simulink model "BMD_2_backup"  (R2025b)
settings: Solver=FixedStepAuto  StartTime=0.0  StopTime=15  FixedStep=0.005  RelTol=1e-3
values from neighbouring files (symbols this model uses):
  FPV_mass = 0.8    [Soft.m]
  g = 9.81    [Soft.m]
  ks = 0    [Soft.m]
  p_0 = 1013.25    [Soft.m]
  Q2Ts = forcetomotors()    [Soft.m]    (also in forcetomotors.m = inv(Ts2Q))
  takeOffDuration = 2    [Soft.m]
  Ts = 0.005    [Soft.m]
undefined symbols (not defined in the file or in its folder): CdA, DiscIntNeverNeededParam, Dw, kd_dz, kd_pos_dx, kd_pos_dy, kd_pq, kd_pr, kd_y, kd_z, ki_dz, ki_pos_dx, ki_pos_dy, ki_pq, ki_pr, ki_y, ki_z, kp_dz, kp_pos_dx, kp_pos_dy, kp_pos_x, kp_pos_y, kp_pq, kp_pr, kp_y, kp_z, pInitialization, rho
libraries: simulink x43, discretizing x18, slpidlib x3, SignalEditorBlockLib x2, shared6dof x1, dynamicsLibrary x1, aerolibasang x1, aerolibnav x1
(part 9 of 22)

== system BMD_2_backup/FCS/Controller/position_controller/pos_dx_pid/Sum ==
  P : Inport  SampleTime=SampleTime
  I : Inport  Port=2  SampleTime=SampleTime
  D : Inport  Port=3  SampleTime=SampleTime
  Passthrough_I : Subsystem  VariantControl=Passthrough_I
  Passthrough_P : Subsystem  VariantControl=Passthrough_P
  Sum_PD : Subsystem  VariantControl=Sum_PD
  Sum_PI : Subsystem  VariantControl=Sum_PI
  Sum_PID : Subsystem  VariantControl=Sum_PID
  Out1 : Outport  SampleTime=SampleTime

== system BMD_2_backup/FCS/Controller/position_controller/pos_dx_pid/Sum Fdbk ==
  fromP : Inport  SampleTime=SampleTime
  fromState : Inport  Port=2  SampleTime=SampleTime
  fromD : Inport  Port=3  SampleTime=SampleTime
  Disabled : Subsystem  VariantControl=Disabled
  Enabled : Subsystem  VariantControl=Enabled
  Passthrough : Subsystem  VariantControl=Passthrough
  Out1 : Outport  SampleTime=SampleTime

== system BMD_2_backup/FCS/Controller/position_controller/pos_dx_pid/Tracking Mode ==
  uout : Inport  SampleTime=SampleTime
  TR : Inport  Port=2  SampleTime=SampleTime
  Disabled : Subsystem  VariantControl=Disabled
  Enabled : Subsystem  VariantControl=Enabled
  Out1 : Outport  SampleTime=SampleTime

== system BMD_2_backup/FCS/Controller/position_controller/pos_dx_pid/Tracking Mode Sum ==
  fromIgain : Inport  SampleTime=SampleTime
  fromTR : Inport  Port=2  SampleTime=SampleTime
  Passthrough : Subsystem  VariantControl=Passthrough
  Tracking Mode : Subsystem  VariantControl=TrackingMode
  preInt : Outport

== system BMD_2_backup/FCS/Controller/position_controller/pos_dx_pid/Tsamp - Integral ==
  U : Inport  SampleTime=SampleTime
  Ts : Inport  Port=2  SampleTime=SampleTime
  Disabled : Subsystem  VariantControl=Disabled
  External Ts : Subsystem  VariantControl=ExternalTs
  Passthrough : Subsystem  VariantControl=Passthrough
  TsSignalSpecification : Subsystem  VariantControl=Disabled_SignalSpec
  Out1 : Outport  SampleTime=SampleTime

== system BMD_2_backup/FCS/Controller/position_controller/pos_dx_pid/Tsamp - Ngain ==
  U : Inport  SampleTime=SampleTime
  Ts : Inport  Port=2  SampleTime=SampleTime
  External Ts : Subsystem  VariantControl=ExternalTs
  Passthrough : Subsystem  VariantControl=Passthrough
  Out1 : Outport  SampleTime=SampleTime

== system BMD_2_backup/FCS/Controller/position_controller/pos_dx_pid/postSat Signal ==
  feedback : Inport  SampleTime=SampleTime
  forward : Inport  Port=2  SampleTime=SampleTime
  Feedback_Path : Subsystem  VariantControl=Feedback
  Forward_Path : Subsystem  VariantControl=Forward
  Out1 : Outport  SampleTime=SampleTime

== system BMD_2_backup/FCS/Controller/position_controller/pos_dx_pid/preInt Signal ==
  preInt : Inport  SampleTime=SampleTime
  extAW : Inport  Port=2  SampleTime=SampleTime
  External PreInt : Subsystem  VariantControl=ExternalPreInt
  Internal PreInt : Subsystem  VariantControl=InternalPreInt
  Out1 : Outport  SampleTime=SampleTime

== system BMD_2_backup/FCS/Controller/position_controller/pos_dx_pid/preSat Signal ==
  feedback : Inport  SampleTime=SampleTime
  forward : Inport  Port=2  SampleTime=SampleTime
  Feedback_Path : Subsystem  VariantControl=Feedback
  Forward_Path : Subsystem  VariantControl=Forward
  Out1 : Outport  SampleTime=SampleTime

== system BMD_2_backup/FCS/Controller/position_controller/pos_dy_pid/Anti-windup ==
  preSat : Inport  SampleTime=SampleTime
  postSat : Inport  Port=2  SampleTime=SampleTime
  P : Inport  Port=3  SampleTime=SampleTime
  preInt : Inport  Port=4  SampleTime=SampleTime
  Upper Limit : Inport  Port=5  SampleTime=SampleTime
  Lower Limit : Inport  Port=6  SampleTime=SampleTime
  Back Calculation : Subsystem  VariantControl=BackCalculation
  Cont. Clamping Ideal : Subsystem  VariantControl=ContClampingIdeal
  Cont. Clamping Parallel : Subsystem  VariantControl=ContClampingParallel
  Disabled : Subsystem  VariantControl=Disabled
  Disc. Clamping Ideal : Subsystem  VariantControl=DiscClampingIdeal
  Disc. Clamping Parallel : Subsystem  VariantControl=DiscClampingParallel
  Passthrough : Subsystem  VariantControl=Passthrough
  Out1 : Outport  SampleTime=SampleTime

== system BMD_2_backup/FCS/Controller/position_controller/pos_dy_pid/D Gain ==
  err : Inport  SampleTime=SampleTime
  D Gain : Inport  Port=2  SampleTime=SampleTime
  Disabled : Subsystem  VariantControl=Disabled
  External Parameters : Subsystem  VariantControl=ExternalParameters
  Internal Parameters : Subsystem  VariantControl=InternalParameters
  Out1 : Outport  SampleTime=SampleTime

== system BMD_2_backup/FCS/Controller/position_controller/pos_dy_pid/External Derivative ==
  err : Inport  SampleTime=SampleTime
  ydot : Inport  Port=2  SampleTime=SampleTime
  Disabled : Subsystem  VariantControl=Disabled
  Error : Subsystem  VariantControl=ErrorSignal
  External Ydot : Subsystem  VariantControl=ExternalYdot
  Out1 : Outport  SampleTime=SampleTime

== system BMD_2_backup/FCS/Controller/position_controller/pos_dy_pid/Filter ==
  Reset : Inport  SampleTime=SampleTime
  U : Inport  Port=2  SampleTime=SampleTime
  N : Inport  Port=3  SampleTime=SampleTime
  D0in : Inport  Port=4  SampleTime=SampleTime
  Nout : Inport  Port=5  SampleTime=SampleTime
  Ts : Inport  Port=6  SampleTime=SampleTime
  Cont. Filter : Subsystem  VariantControl=ContFilter
  Cont. Filter Only : Subsystem  VariantControl=ContFilterOnly
  Differentiator : Subsystem  VariantControl=Differentiator
  Disabled : Subsystem  VariantControl=Disabled
  Disc. Backward Euler Filter : Subsystem  VariantControl=BackwardEulerFilter
  Disc. Backward Euler Filter Only : Subsystem  VariantControl=BackwardEulerFilterOnly
  Disc. Forward Euler Filter : Subsystem  VariantControl=ForwardEulerFilter
  Disc. Forward Euler Filter Only : Subsystem  VariantControl=ForwardEulerFilterOnly
  Disc. Trapezoidal Filter : Subsystem  VariantControl=TrapezoidalFilter
  Disc. Trapezoidal Filter Only : Subsystem  VariantControl=TrapezoidalFilterOnly
  Passthrough : Subsystem  VariantControl=Passthrough
  Y : Outport  SampleTime=SampleTime

== system BMD_2_backup/FCS/Controller/position_controller/pos_dy_pid/Filter ICs ==
  D0 : Inport  SampleTime=SampleTime
  Disabled : Subsystem  VariantControl=Disabled
  External IC : Subsystem  VariantControl=ExternalICs
  Internal IC - Differentiator : Subsystem  VariantControl=InternalICsDifferentiator
  Internal IC - Filter : Subsystem  VariantControl=InternalICsFilter
  Out1 : Outport  SampleTime=SampleTime

== system BMD_2_backup/FCS/Controller/position_controller/pos_dy_pid/I Gain ==
  err : Inport  SampleTime=SampleTime
  I Gain : Inport  Port=2  SampleTime=SampleTime
  Disabled : Subsystem  VariantControl=Disabled
  External Parameters : Subsystem  VariantControl=ExternalParameters
  Internal Parameters : Subsystem  VariantControl=InternalParameters
  Out1 : Outport  SampleTime=SampleTime

== system BMD_2_backup/FCS/Controller/position_controller/pos_dy_pid/Ideal P Gain ==
  In1 : Inport  SampleTime=SampleTime
  P Gain : Inport  Port=2  SampleTime=SampleTime
  External Parameters : Subsystem  VariantControl=ExternalParameters
  Internal Parameters : Subsystem  VariantControl=InternalParameters
  Passthrough : Subsystem  VariantControl=Disabled
  Out1 : Outport  SampleTime=SampleTime

== system BMD_2_backup/FCS/Controller/position_controller/pos_dy_pid/Ideal P Gain Fdbk ==
  In1 : Inport  SampleTime=SampleTime
  P Gain : Inport  Port=2  SampleTime=SampleTime
  Disabled : Subsystem  VariantControl=Disabled
  External Parameters : Subsystem  VariantControl=ExternalParameters
  Internal Parameters : Subsystem  VariantControl=InternalParameters
  Passthrough : Subsystem  VariantControl=Passthrough
  Out1 : Outport  SampleTime=SampleTime

== system BMD_2_backup/FCS/Controller/position_controller/pos_dy_pid/Integrator ==
  U : Inport  SampleTime=SampleTime
  I0in : Inport  Port=2  SampleTime=SampleTime
  Reset : Inport  Port=3  SampleTime=SampleTime
  Continuous : Subsystem  VariantControl=Continuous
  Disabled : Subsystem  VariantControl=Disabled
  Discrete : Subsystem  VariantControl=Discrete
  state : Outport  SampleTime=SampleTime
  out : Outport  Port=2  SampleTime=SampleTime

== system BMD_2_backup/FCS/Controller/position_controller/pos_dy_pid/Integrator ICs ==
  I0 : Inport  SampleTime=SampleTime
  Disabled : Subsystem  VariantControl=Disabled
  External IC : Subsystem  VariantControl=ExternalICs
  Internal IC : Subsystem  VariantControl=InternalICs
  Out1 : Outport  SampleTime=SampleTime

== system BMD_2_backup/FCS/Controller/position_controller/pos_dy_pid/N Copy ==
  N Gain : Inport  SampleTime=SampleTime
  Disabled : Subsystem  VariantControl=Disabled
  Disabled wSignal Specification : Subsystem  VariantControl=Disabled_SignalSpec
  External Parameters : Subsystem  VariantControl=ExternalParameters
  Internal Parameters : Subsystem  VariantControl=InternalParameters
  Out1 : Outport  SampleTime=SampleTime

== system BMD_2_backup/FCS/Controller/position_controller/pos_dy_pid/N Gain ==
  U : Inport  SampleTime=SampleTime
  N Gain : Inport  Port=2  SampleTime=SampleTime
  Disabled : Subsystem  VariantControl=Disabled
  External Parameters : Subsystem  VariantControl=ExternalParameters
  Internal Parameters : Subsystem  VariantControl=InternalParameters
  Passthrough : Subsystem  VariantControl=Passthrough
  Out1 : Outport  SampleTime=SampleTime

== system BMD_2_backup/FCS/Controller/position_controller/pos_dy_pid/P Copy ==
  P Gain : Inport  SampleTime=SampleTime
  Disabled : Subsystem  VariantControl=Disabled
  External Parameters Ideal : Subsystem  VariantControl=ExternalParamsIdeal
  Internal Parameters Ideal : Subsystem  VariantControl=InternalParamsIdeal
  Out1 : Outport  SampleTime=SampleTime

== system BMD_2_backup/FCS/Controller/position_controller/pos_dy_pid/PID Compensator Formula ==

== system BMD_2_backup/FCS/Controller/position_controller/pos_dy_pid/Parallel P Gain ==
  err : Inport  SampleTime=SampleTime
  P Gain : Inport  Port=2  SampleTime=SampleTime
  Disabled : Subsystem  VariantControl=Disabled
  External Parameters : Subsystem  VariantControl=ExternalParameters
  Internal Parameters : Subsystem  VariantControl=InternalParameters
  Passthrough : Subsystem  VariantControl=Passthrough
  Out1 : Outport  SampleTime=SampleTime

== system BMD_2_backup/FCS/Controller/position_controller/pos_dy_pid/Reset Signal ==
  Reset : Inport  SampleTime=SampleTime
  Disabled : Subsystem  VariantControl=Disabled
  External Reset : Subsystem  VariantControl=ExternalReset
  Out1 : Outport  SampleTime=SampleTime

== system BMD_2_backup/FCS/Controller/position_controller/pos_dy_pid/Saturation ==
  In1 : Inport  SampleTime=SampleTime
  Upper Limit : Inport  Port=2  SampleTime=SampleTime
  Lower Limit : Inport  Port=3  SampleTime=SampleTime
  Enabled : Subsystem  VariantControl=Enabled
  External : Subsystem  VariantControl=External
  Passthrough : Subsystem  VariantControl=Disabled
  Out1 : Outport  SampleTime=SampleTime

== system BMD_2_backup/FCS/Controller/position_controller/pos_dy_pid/Saturation Fdbk ==
  In1 : Inport  SampleTime=SampleTime
  Upper Limit : Inport  Port=2  SampleTime=SampleTime
  Lower Limit : Inport  Port=3  SampleTime=SampleTime
  Disabled : Subsystem  VariantControl=Disabled
  Enabled : Subsystem  VariantControl=Enabled
  External : Subsystem  VariantControl=External
  Passthrough : Subsystem  VariantControl=Passthrough
  Out1 : Outport  SampleTime=SampleTime

== system BMD_2_backup/FCS/Controller/position_controller/pos_dy_pid/Sum ==
  P : Inport  SampleTime=SampleTime
  I : Inport  Port=2  SampleTime=SampleTime
  D : Inport  Port=3  SampleTime=SampleTime
  Passthrough_I : Subsystem  VariantControl=Passthrough_I
  Passthrough_P : Subsystem  VariantControl=Passthrough_P
  Sum_PD : Subsystem  VariantControl=Sum_PD
  Sum_PI : Subsystem  VariantControl=Sum_PI
  Sum_PID : Subsystem  VariantControl=Sum_PID
  Out1 : Outport  SampleTime=SampleTime

== system BMD_2_backup/FCS/Controller/position_controller/pos_dy_pid/Sum Fdbk ==
  fromP : Inport  SampleTime=SampleTime
  fromState : Inport  Port=2  SampleTime=SampleTime
  fromD : Inport  Port=3  SampleTime=SampleTime
  Disabled : Subsystem  VariantControl=Disabled
  Enabled : Subsystem  VariantControl=Enabled
  Passthrough : Subsystem  VariantControl=Passthrough
  Out1 : Outport  SampleTime=SampleTime

== system BMD_2_backup/FCS/Controller/position_controller/pos_dy_pid/Tracking Mode ==
  uout : Inport  SampleTime=SampleTime
  TR : Inport  Port=2  SampleTime=SampleTime
  Disabled : Subsystem  VariantControl=Disabled
  Enabled : Subsystem  VariantControl=Enabled
  Out1 : Outport  SampleTime=SampleTime

== system BMD_2_backup/FCS/Controller/position_controller/pos_dy_pid/Tracking Mode Sum ==
  fromIgain : Inport  SampleTime=SampleTime
  fromTR : Inport  Port=2  SampleTime=SampleTime
  Passthrough : Subsystem  VariantControl=Passthrough
  Tracking Mode : Subsystem  VariantControl=TrackingMode
  preInt : Outport

== system BMD_2_backup/FCS/Controller/position_controller/pos_dy_pid/Tsamp - Integral ==
  U : Inport  SampleTime=SampleTime
  Ts : Inport  Port=2  SampleTime=SampleTime
  Disabled : Subsystem  VariantControl=Disabled
  External Ts : Subsystem  VariantControl=ExternalTs
  Passthrough : Subsystem  VariantControl=Passthrough
  TsSignalSpecification : Subsystem  VariantControl=Disabled_SignalSpec
  Out1 : Outport  SampleTime=SampleTime

== system BMD_2_backup/FCS/Controller/position_controller/pos_dy_pid/Tsamp - Ngain ==
  U : Inport  SampleTime=SampleTime
  Ts : Inport  Port=2  SampleTime=SampleTime
  External Ts : Subsystem  VariantControl=ExternalTs
  Passthrough : Subsystem  VariantControl=Passthrough
  Out1 : Outport  SampleTime=SampleTime

== system BMD_2_backup/FCS/Controller/position_controller/pos_dy_pid/postSat Signal ==
  feedback : Inport  SampleTime=SampleTime
  forward : Inport  Port=2  SampleTime=SampleTime
  Feedback_Path : Subsystem  VariantControl=Feedback
  Forward_Path : Subsystem  VariantControl=Forward
  Out1 : Outport  SampleTime=SampleTime

== system BMD_2_backup/FCS/Controller/position_controller/pos_dy_pid/preInt Signal ==
  preInt : Inport  SampleTime=SampleTime
  extAW : Inport  Port=2  SampleTime=SampleTime
  External PreInt : Subsystem  VariantControl=ExternalPreInt
  Internal PreInt : Subsystem  VariantControl=InternalPreInt
  Out1 : Outport  SampleTime=SampleTime

== system BMD_2_backup/FCS/Controller/position_controller/pos_dy_pid/preSat Signal ==
  feedback : Inport  SampleTime=SampleTime
  forward : Inport  Port=2  SampleTime=SampleTime
  Feedback_Path : Subsystem  VariantControl=Feedback
  Forward_Path : Subsystem  VariantControl=Forward
  Out1 : Outport  SampleTime=SampleTime

== system BMD_2_backup/FCS/Controller/position_controller/pos_x_pid/Anti-windup ==
  preSat : Inport  SampleTime=SampleTime
  postSat : Inport  Port=2  SampleTime=SampleTime
  P : Inport  Port=3  SampleTime=SampleTime
  preInt : Inport  Port=4  SampleTime=SampleTime
  Upper Limit : Inport  Port=5  SampleTime=SampleTime
  Lower Limit : Inport  Port=6  SampleTime=SampleTime
  Back Calculation : Subsystem  VariantControl=BackCalculation
  Cont. Clamping Ideal : Subsystem  VariantControl=ContClampingIdeal
  Cont. Clamping Parallel : Subsystem  VariantControl=ContClampingParallel
  Disabled : Subsystem  VariantControl=Disabled
  Disc. Clamping Ideal : Subsystem  VariantControl=DiscClampingIdeal
  Disc. Clamping Parallel : Subsystem  VariantControl=DiscClampingParallel
  Passthrough : Subsystem  VariantControl=Passthrough
  Out1 : Outport  SampleTime=SampleTime

== system BMD_2_backup/FCS/Controller/position_controller/pos_x_pid/D Gain ==
  err : Inport  SampleTime=SampleTime
  D Gain : Inport  Port=2  SampleTime=SampleTime
  Disabled : Subsystem  VariantControl=Disabled
  External Parameters : Subsystem  VariantControl=ExternalParameters
  Internal Parameters : Subsystem  VariantControl=InternalParameters
  Out1 : Outport  SampleTime=SampleTime

== system BMD_2_backup/FCS/Controller/position_controller/pos_x_pid/External Derivative ==
  err : Inport  SampleTime=SampleTime
  ydot : Inport  Port=2  SampleTime=SampleTime
  Disabled : Subsystem  VariantControl=Disabled
  Error : Subsystem  VariantControl=ErrorSignal
  External Ydot : Subsystem  VariantControl=ExternalYdot
  Out1 : Outport  SampleTime=SampleTime

== system BMD_2_backup/FCS/Controller/position_controller/pos_x_pid/Filter ==
  Reset : Inport  SampleTime=SampleTime
  U : Inport  Port=2  SampleTime=SampleTime
  N : Inport  Port=3  SampleTime=SampleTime
  D0in : Inport  Port=4  SampleTime=SampleTime
  Nout : Inport  Port=5  SampleTime=SampleTime
  Ts : Inport  Port=6  SampleTime=SampleTime
  Cont. Filter : Subsystem  VariantControl=ContFilter
  Cont. Filter Only : Subsystem  VariantControl=ContFilterOnly
  Differentiator : Subsystem  VariantControl=Differentiator
  Disabled : Subsystem  VariantControl=Disabled
  Disc. Backward Euler Filter : Subsystem  VariantControl=BackwardEulerFilter
  Disc. Backward Euler Filter Only : Subsystem  VariantControl=BackwardEulerFilterOnly
  Disc. Forward Euler Filter : Subsystem  VariantControl=ForwardEulerFilter
  Disc. Forward Euler Filter Only : Subsystem  VariantControl=ForwardEulerFilterOnly
  Disc. Trapezoidal Filter : Subsystem  VariantControl=TrapezoidalFilter
  Disc. Trapezoidal Filter Only : Subsystem  VariantControl=TrapezoidalFilterOnly
  Passthrough : Subsystem  VariantControl=Passthrough
  Y : Outport  SampleTime=SampleTime

== system BMD_2_backup/FCS/Controller/position_controller/pos_x_pid/Filter ICs ==
  D0 : Inport  SampleTime=SampleTime
  Disabled : Subsystem  VariantControl=Disabled
  External IC : Subsystem  VariantControl=ExternalICs
  Internal IC - Differentiator : Subsystem  VariantControl=InternalICsDifferentiator
  Internal IC - Filter : Subsystem  VariantControl=InternalICsFilter
  Out1 : Outport  SampleTime=SampleTime

== system BMD_2_backup/FCS/Controller/position_controller/pos_x_pid/I Gain ==
  err : Inport  SampleTime=SampleTime
  I Gain : Inport  Port=2  SampleTime=SampleTime
  Disabled : Subsystem  VariantControl=Disabled
  External Parameters : Subsystem  VariantControl=ExternalParameters
  Internal Parameters : Subsystem  VariantControl=InternalParameters
  Out1 : Outport  SampleTime=SampleTime

== system BMD_2_backup/FCS/Controller/position_controller/pos_x_pid/Ideal P Gain ==
  In1 : Inport  SampleTime=SampleTime
  P Gain : Inport  Port=2  SampleTime=SampleTime
  External Parameters : Subsystem  VariantControl=ExternalParameters
  Internal Parameters : Subsystem  VariantControl=InternalParameters
  Passthrough : Subsystem  VariantControl=Disabled
  Out1 : Outport  SampleTime=SampleTime

== system BMD_2_backup/FCS/Controller/position_controller/pos_x_pid/Ideal P Gain Fdbk ==
  In1 : Inport  SampleTime=SampleTime
  P Gain : Inport  Port=2  SampleTime=SampleTime
  Disabled : Subsystem  VariantControl=Disabled
  External Parameters : Subsystem  VariantControl=ExternalParameters
  Internal Parameters : Subsystem  VariantControl=InternalParameters
  Passthrough : Subsystem  VariantControl=Passthrough
  Out1 : Outport  SampleTime=SampleTime

== system BMD_2_backup/FCS/Controller/position_controller/pos_x_pid/Integrator ==
  U : Inport  SampleTime=SampleTime
  I0in : Inport  Port=2  SampleTime=SampleTime
  Reset : Inport  Port=3  SampleTime=SampleTime
  Continuous : Subsystem  VariantControl=Continuous
  Disabled : Subsystem  VariantControl=Disabled
  Discrete : Subsystem  VariantControl=Discrete
  state : Outport  SampleTime=SampleTime
  out : Outport  Port=2  SampleTime=SampleTime

== system BMD_2_backup/FCS/Controller/position_controller/pos_x_pid/Integrator ICs ==
  I0 : Inport  SampleTime=SampleTime
  Disabled : Subsystem  VariantControl=Disabled
  External IC : Subsystem  VariantControl=ExternalICs
  Internal IC : Subsystem  VariantControl=InternalICs
  Out1 : Outport  SampleTime=SampleTime

== system BMD_2_backup/FCS/Controller/position_controller/pos_x_pid/N Copy ==
  N Gain : Inport  SampleTime=SampleTime
  Disabled : Subsystem  VariantControl=Disabled
  Disabled wSignal Specification : Subsystem  VariantControl=Disabled_SignalSpec
  External Parameters : Subsystem  VariantControl=ExternalParameters
  Internal Parameters : Subsystem  VariantControl=InternalParameters
  Out1 : Outport  SampleTime=SampleTime

== system BMD_2_backup/FCS/Controller/position_controller/pos_x_pid/N Gain ==
  U : Inport  SampleTime=SampleTime
  N Gain : Inport  Port=2  SampleTime=SampleTime
  Disabled : Subsystem  VariantControl=Disabled
  External Parameters : Subsystem  VariantControl=ExternalParameters
  Internal Parameters : Subsystem  VariantControl=InternalParameters
  Passthrough : Subsystem  VariantControl=Passthrough
  Out1 : Outport  SampleTime=SampleTime

== system BMD_2_backup/FCS/Controller/position_controller/pos_x_pid/P Copy ==
  P Gain : Inport  SampleTime=SampleTime
  Disabled : Subsystem  VariantControl=Disabled
  External Parameters Ideal : Subsystem  VariantControl=ExternalParamsIdeal
  Internal Parameters Ideal : Subsystem  VariantControl=InternalParamsIdeal
  Out1 : Outport  SampleTime=SampleTime

== system BMD_2_backup/FCS/Controller/position_controller/pos_x_pid/PID Compensator Formula ==

== system BMD_2_backup/FCS/Controller/position_controller/pos_x_pid/Parallel P Gain ==
  err : Inport  SampleTime=SampleTime
  P Gain : Inport  Port=2  SampleTime=SampleTime
  Disabled : Subsystem  VariantControl=Disabled
  External Parameters : Subsystem  VariantControl=ExternalParameters
  Internal Parameters : Subsystem  VariantControl=InternalParameters
  Passthrough : Subsystem  VariantControl=Passthrough
  Out1 : Outport  SampleTime=SampleTime

== system BMD_2_backup/FCS/Controller/position_controller/pos_x_pid/Reset Signal ==
  Reset : Inport  SampleTime=SampleTime
  Disabled : Subsystem  VariantControl=Disabled
  External Reset : Subsystem  VariantControl=ExternalReset
  Out1 : Outport  SampleTime=SampleTime

== system BMD_2_backup/FCS/Controller/position_controller/pos_x_pid/Saturation ==
  In1 : Inport  SampleTime=SampleTime
  Upper Limit : Inport  Port=2  SampleTime=SampleTime
  Lower Limit : Inport  Port=3  SampleTime=SampleTime
  Enabled : Subsystem  VariantControl=Enabled
  External : Subsystem  VariantControl=External
  Passthrough : Subsystem  VariantControl=Disabled
  Out1 : Outport  SampleTime=SampleTime

== system BMD_2_backup/FCS/Controller/position_controller/pos_x_pid/Saturation Fdbk ==
  In1 : Inport  SampleTime=SampleTime
  Upper Limit : Inport  Port=2  SampleTime=SampleTime
  Lower Limit : Inport  Port=3  SampleTime=SampleTime
  Disabled : Subsystem  VariantControl=Disabled
  Enabled : Subsystem  VariantControl=Enabled
  External : Subsystem  VariantControl=External
  Passthrough : Subsystem  VariantControl=Passthrough
  Out1 : Outport  SampleTime=SampleTime

== system BMD_2_backup/FCS/Controller/position_controller/pos_x_pid/Sum ==
  P : Inport  SampleTime=SampleTime
  I : Inport  Port=2  SampleTime=SampleTime
  D : Inport  Port=3  SampleTime=SampleTime
  Passthrough_I : Subsystem  VariantControl=Passthrough_I
  Passthrough_P : Subsystem  VariantControl=Passthrough_P
  Sum_PD : Subsystem  VariantControl=Sum_PD
  Sum_PI : Subsystem  VariantControl=Sum_PI
  Sum_PID : Subsystem  VariantControl=Sum_PID
  Out1 : Outport  SampleTime=SampleTime

== system BMD_2_backup/FCS/Controller/position_controller/pos_x_pid/Sum Fdbk ==
  fromP : Inport  SampleTime=SampleTime
  fromState : Inport  Port=2  SampleTime=SampleTime
  fromD : Inport  Port=3  SampleTime=SampleTime
  Disabled : Subsystem  VariantControl=Disabled
  Enabled : Subsystem  VariantControl=Enabled
  Passthrough : Subsystem  VariantControl=Passthrough
  Out1 : Outport  SampleTime=SampleTime

== system BMD_2_backup/FCS/Controller/position_controller/pos_x_pid/Tracking Mode ==
  uout : Inport  SampleTime=SampleTime
  TR : Inport  Port=2  SampleTime=SampleTime
  Disabled : Subsystem  VariantControl=Disabled
  Enabled : Subsystem  VariantControl=Enabled
  Out1 : Outport  SampleTime=SampleTime

== system BMD_2_backup/FCS/Controller/position_controller/pos_x_pid/Tracking Mode Sum ==
  fromIgain : Inport  SampleTime=SampleTime
  fromTR : Inport  Port=2  SampleTime=SampleTime
  Passthrough : Subsystem  VariantControl=Passthrough
  Tracking Mode : Subsystem  VariantControl=TrackingMode
  preInt : Outport

== system BMD_2_backup/FCS/Controller/position_controller/pos_x_pid/Tsamp - Integral ==
  U : Inport  SampleTime=SampleTime
  Ts : Inport  Port=2  SampleTime=SampleTime
  Disabled : Subsystem  VariantControl=Disabled
  External Ts : Subsystem  VariantControl=ExternalTs
  Passthrough : Subsystem  VariantControl=Passthrough
  TsSignalSpecification : Subsystem  VariantControl=Disabled_SignalSpec
  Out1 : Outport  SampleTime=SampleTime

== system BMD_2_backup/FCS/Controller/position_controller/pos_x_pid/Tsamp - Ngain ==
  U : Inport  SampleTime=SampleTime
  Ts : Inport  Port=2  SampleTime=SampleTime
  External Ts : Subsystem  VariantControl=ExternalTs
  Passthrough : Subsystem  VariantControl=Passthrough
  Out1 : Outport  SampleTime=SampleTime

== system BMD_2_backup/FCS/Controller/position_controller/pos_x_pid/postSat Signal ==
  feedback : Inport  SampleTime=SampleTime
  forward : Inport  Port=2  SampleTime=SampleTime
  Feedback_Path : Subsystem  VariantControl=Feedback
  Forward_Path : Subsystem  VariantControl=Forward
  Out1 : Outport  SampleTime=SampleTime

== system BMD_2_backup/FCS/Controller/position_controller/pos_x_pid/preInt Signal ==
  preInt : Inport  SampleTime=SampleTime
  extAW : Inport  Port=2  SampleTime=SampleTime
  External PreInt : Subsystem  VariantControl=ExternalPreInt
  Internal PreInt : Subsystem  VariantControl=InternalPreInt
  Out1 : Outport  SampleTime=SampleTime

== system BMD_2_backup/FCS/Controller/position_controller/pos_x_pid/preSat Signal ==
  feedback : Inport  SampleTime=SampleTime
  forward : Inport  Port=2  SampleTime=SampleTime
  Feedback_Path : Subsystem  VariantControl=Feedback
  Forward_Path : Subsystem  VariantControl=Forward
  Out1 : Outport  SampleTime=SampleTime

== system BMD_2_backup/FCS/Controller/position_controller/pos_y_pid/Anti-windup ==
  preSat : Inport  SampleTime=SampleTime
  postSat : Inport  Port=2  SampleTime=SampleTime
  P : Inport  Port=3  SampleTime=SampleTime
  preInt : Inport  Port=4  SampleTime=SampleTime
  Upper Limit : Inport  Port=5  SampleTime=SampleTime
  Lower Limit : Inport  Port=6  SampleTime=SampleTime
  Back Calculation : Subsystem  VariantControl=BackCalculation
  Cont. Clamping Ideal : Subsystem  VariantControl=ContClampingIdeal
  Cont. Clamping Parallel : Subsystem  VariantControl=ContClampingParallel
  Disabled : Subsystem  VariantControl=Disabled
  Disc. Clamping Ideal : Subsystem  VariantControl=DiscClampingIdeal
  Disc. Clamping Parallel : Subsystem  VariantControl=DiscClampingParallel
  Passthrough : Subsystem  VariantControl=Passthrough
  Out1 : Outport  SampleTime=SampleTime

== system BMD_2_backup/FCS/Controller/position_controller/pos_y_pid/D Gain ==
  err : Inport  SampleTime=SampleTime
  D Gain : Inport  Port=2  SampleTime=SampleTime
  Disabled : Subsystem  VariantControl=Disabled
  External Parameters : Subsystem  VariantControl=ExternalParameters
  Internal Parameters : Subsystem  VariantControl=InternalParameters
  Out1 : Outport  SampleTime=SampleTime

== system BMD_2_backup/FCS/Controller/position_controller/pos_y_pid/External Derivative ==
  err : Inport  SampleTime=SampleTime
  ydot : Inport  Port=2  SampleTime=SampleTime
  Disabled : Subsystem  VariantControl=Disabled
  Error : Subsystem  VariantControl=ErrorSignal
  External Ydot : Subsystem  VariantControl=ExternalYdot
  Out1 : Outport  SampleTime=SampleTime

== system BMD_2_backup/FCS/Controller/position_controller/pos_y_pid/Filter ==
  Reset : Inport  SampleTime=SampleTime
  U : Inport  Port=2  SampleTime=SampleTime
  N : Inport  Port=3  SampleTime=SampleTime
  D0in : Inport  Port=4  SampleTime=SampleTime
  Nout : Inport  Port=5  SampleTime=SampleTime
  Ts : Inport  Port=6  SampleTime=SampleTime
  Cont. Filter : Subsystem  VariantControl=ContFilter
  Cont. Filter Only : Subsystem  VariantControl=ContFilterOnly
  Differentiator : Subsystem  VariantControl=Differentiator
  Disabled : Subsystem  VariantControl=Disabled
  Disc. Backward Euler Filter : Subsystem  VariantControl=BackwardEulerFilter
  Disc. Backward Euler Filter Only : Subsystem  VariantControl=BackwardEulerFilterOnly
  Disc. Forward Euler Filter : Subsystem  VariantControl=ForwardEulerFilter
  Disc. Forward Euler Filter Only : Subsystem  VariantControl=ForwardEulerFilterOnly
  Disc. Trapezoidal Filter : Subsystem  VariantControl=TrapezoidalFilter
  Disc. Trapezoidal Filter Only : Subsystem  VariantControl=TrapezoidalFilterOnly
  Passthrough : Subsystem  VariantControl=Passthrough
  Y : Outport  SampleTime=SampleTime

== system BMD_2_backup/FCS/Controller/position_controller/pos_y_pid/Filter ICs ==
  D0 : Inport  SampleTime=SampleTime
  Disabled : Subsystem  VariantControl=Disabled
  External IC : Subsystem  VariantControl=ExternalICs
  Internal IC - Differentiator : Subsystem  VariantControl=InternalICsDifferentiator
  Internal IC - Filter : Subsystem  VariantControl=InternalICsFilter
  Out1 : Outport  SampleTime=SampleTime

== system BMD_2_backup/FCS/Controller/position_controller/pos_y_pid/I Gain ==
  err : Inport  SampleTime=SampleTime
  I Gain : Inport  Port=2  SampleTime=SampleTime
  Disabled : Subsystem  VariantControl=Disabled
  External Parameters : Subsystem  VariantControl=ExternalParameters
  Internal Parameters : Subsystem  VariantControl=InternalParameters
  Out1 : Outport  SampleTime=SampleTime

== system BMD_2_backup/FCS/Controller/position_controller/pos_y_pid/Ideal P Gain ==
  In1 : Inport  SampleTime=SampleTime
  P Gain : Inport  Port=2  SampleTime=SampleTime
  External Parameters : Subsystem  VariantControl=ExternalParameters
  Internal Parameters : Subsystem  VariantControl=InternalParameters
  Passthrough : Subsystem  VariantControl=Disabled
  Out1 : Outport  SampleTime=SampleTime

== system BMD_2_backup/FCS/Controller/position_controller/pos_y_pid/Ideal P Gain Fdbk ==
  In1 : Inport  SampleTime=SampleTime
  P Gain : Inport  Port=2  SampleTime=SampleTime
  Disabled : Subsystem  VariantControl=Disabled
  External Parameters : Subsystem  VariantControl=ExternalParameters
  Internal Parameters : Subsystem  VariantControl=InternalParameters
  Passthrough : Subsystem  VariantControl=Passthrough
  Out1 : Outport  SampleTime=SampleTime

== system BMD_2_backup/FCS/Controller/position_controller/pos_y_pid/Integrator ==
  U : Inport  SampleTime=SampleTime
  I0in : Inport  Port=2  SampleTime=SampleTime
  Reset : Inport  Port=3  SampleTime=SampleTime
  Continuous : Subsystem  VariantControl=Continuous
  Disabled : Subsystem  VariantControl=Disabled
  Discrete : Subsystem  VariantControl=Discrete
  state : Outport  SampleTime=SampleTime
  out : Outport  Port=2  SampleTime=SampleTime

== system BMD_2_backup/FCS/Controller/position_controller/pos_y_pid/Integrator ICs ==
  I0 : Inport  SampleTime=SampleTime
  Disabled : Subsystem  VariantControl=Disabled
  External IC : Subsystem  VariantControl=ExternalICs
  Internal IC : Subsystem  VariantControl=InternalICs
  Out1 : Outport  SampleTime=SampleTime

== system BMD_2_backup/FCS/Controller/position_controller/pos_y_pid/N Copy ==
  N Gain : Inport  SampleTime=SampleTime
  Disabled : Subsystem  VariantControl=Disabled
  Disabled wSignal Specification : Subsystem  VariantControl=Disabled_SignalSpec
  External Parameters : Subsystem  VariantControl=ExternalParameters
  Internal Parameters : Subsystem  VariantControl=InternalParameters
  Out1 : Outport  SampleTime=SampleTime

== system BMD_2_backup/FCS/Controller/position_controller/pos_y_pid/N Gain ==
  U : Inport  SampleTime=SampleTime
  N Gain : Inport  Port=2  SampleTime=SampleTime
  Disabled : Subsystem  VariantControl=Disabled
  External Parameters : Subsystem  VariantControl=ExternalParameters
  Internal Parameters : Subsystem  VariantControl=InternalParameters
  Passthrough : Subsystem  VariantControl=Passthrough
  Out1 : Outport  SampleTime=SampleTime

== system BMD_2_backup/FCS/Controller/position_controller/pos_y_pid/P Copy ==
  P Gain : Inport  SampleTime=SampleTime
  Disabled : Subsystem  VariantControl=Disabled
  External Parameters Ideal : Subsystem  VariantControl=ExternalParamsIdeal
  Internal Parameters Ideal : Subsystem  VariantControl=InternalParamsIdeal
  Out1 : Outport  SampleTime=SampleTime

== system BMD_2_backup/FCS/Controller/position_controller/pos_y_pid/PID Compensator Formula ==

== system BMD_2_backup/FCS/Controller/position_controller/pos_y_pid/Parallel P Gain ==
  err : Inport  SampleTime=SampleTime
  P Gain : Inport  Port=2  SampleTime=SampleTime
  Disabled : Subsystem  VariantControl=Disabled
  External Parameters : Subsystem  VariantControl=ExternalParameters
  Internal Parameters : Subsystem  VariantControl=InternalParameters
  Passthrough : Subsystem  VariantControl=Passthrough
  Out1 : Outport  SampleTime=SampleTime

== system BMD_2_backup/FCS/Controller/position_controller/pos_y_pid/Reset Signal ==
  Reset : Inport  SampleTime=SampleTime
  Disabled : Subsystem  VariantControl=Disabled
  External Reset : Subsystem  VariantControl=ExternalReset
  Out1 : Outport  SampleTime=SampleTime

== system BMD_2_backup/FCS/Controller/position_controller/pos_y_pid/Saturation ==
  In1 : Inport  SampleTime=SampleTime
  Upper Limit : Inport  Port=2  SampleTime=SampleTime
  Lower Limit : Inport  Port=3  SampleTime=SampleTime
  Enabled : Subsystem  VariantControl=Enabled
  External : Subsystem  VariantControl=External
  Passthrough : Subsystem  VariantControl=Disabled
  Out1 : Outport  SampleTime=SampleTime

== system BMD_2_backup/FCS/Controller/position_controller/pos_y_pid/Saturation Fdbk ==
  In1 : Inport  SampleTime=SampleTime
  Upper Limit : Inport  Port=2  SampleTime=SampleTime
  Lower Limit : Inport  Port=3  SampleTime=SampleTime
  Disabled : Subsystem  VariantControl=Disabled
  Enabled : Subsystem  VariantControl=Enabled
  External : Subsystem  VariantControl=External
  Passthrough : Subsystem  VariantControl=Passthrough
  Out1 : Outport  SampleTime=SampleTime

== system BMD_2_backup/FCS/Controller/position_controller/pos_y_pid/Sum ==
  P : Inport  SampleTime=SampleTime
  I : Inport  Port=2  SampleTime=SampleTime
  D : Inport  Port=3  SampleTime=SampleTime
  Passthrough_I : Subsystem  VariantControl=Passthrough_I
  Passthrough_P : Subsystem  VariantControl=Passthrough_P
  Sum_PD : Subsystem  VariantControl=Sum_PD
  Sum_PI : Subsystem  VariantControl=Sum_PI
  Sum_PID : Subsystem  VariantControl=Sum_PID
  Out1 : Outport  SampleTime=SampleTime

== system BMD_2_backup/FCS/Controller/position_controller/pos_y_pid/Sum Fdbk ==
  fromP : Inport  SampleTime=SampleTime
  fromState : Inport  Port=2  SampleTime=SampleTime
  fromD : Inport  Port=3  SampleTime=SampleTime
  Disabled : Subsystem  VariantControl=Disabled
  Enabled : Subsystem  VariantControl=Enabled
  Passthrough : Subsystem  VariantControl=Passthrough
  Out1 : Outport  SampleTime=SampleTime

== system BMD_2_backup/FCS/Controller/position_controller/pos_y_pid/Tracking Mode ==
  uout : Inport  SampleTime=SampleTime
  TR : Inport  Port=2  SampleTime=SampleTime
  Disabled : Subsystem  VariantControl=Disabled
  Enabled : Subsystem  VariantControl=Enabled
  Out1 : Outport  SampleTime=SampleTime

== system BMD_2_backup/FCS/Controller/position_controller/pos_y_pid/Tracking Mode Sum ==
  fromIgain : Inport  SampleTime=SampleTime
  fromTR : Inport  Port=2  SampleTime=SampleTime
  Passthrough : Subsystem  VariantControl=Passthrough
  Tracking Mode : Subsystem  VariantControl=TrackingMode
  preInt : Outport

== system BMD_2_backup/FCS/Controller/position_controller/pos_y_pid/Tsamp - Integral ==
  U : Inport  SampleTime=SampleTime
  Ts : Inport  Port=2  SampleTime=SampleTime
  Disabled : Subsystem  VariantControl=Disabled
  External Ts : Subsystem  VariantControl=ExternalTs
  Passthrough : Subsystem  VariantControl=Passthrough
  TsSignalSpecification : Subsystem  VariantControl=Disabled_SignalSpec
  Out1 : Outport  SampleTime=SampleTime

== system BMD_2_backup/FCS/Controller/position_controller/pos_y_pid/Tsamp - Ngain ==
  U : Inport  SampleTime=SampleTime
  Ts : Inport  Port=2  SampleTime=SampleTime
  External Ts : Subsystem  VariantControl=ExternalTs
  Passthrough : Subsystem  VariantControl=Passthrough
  Out1 : Outport  SampleTime=SampleTime

== system BMD_2_backup/FCS/Controller/position_controller/pos_y_pid/postSat Signal ==
  feedback : Inport  SampleTime=SampleTime
  forward : Inport  Port=2  SampleTime=SampleTime
  Feedback_Path : Subsystem  VariantControl=Feedback
  Forward_Path : Subsystem  VariantControl=Forward
  Out1 : Outport  SampleTime=SampleTime

== system BMD_2_backup/FCS/Controller/position_controller/pos_y_pid/preInt Signal ==
  preInt : Inport  SampleTime=SampleTime
  extAW : Inport  Port=2  SampleTime=SampleTime
  External PreInt : Subsystem  VariantControl=ExternalPreInt
  Internal PreInt : Subsystem  VariantControl=InternalPreInt
  Out1 : Outport  SampleTime=SampleTime

== system BMD_2_backup/FCS/Controller/position_controller/pos_y_pid/preSat Signal ==
  feedback : Inport  SampleTime=SampleTime
  forward : Inport  Port=2  SampleTime=SampleTime
  Feedback_Path : Subsystem  VariantControl=Feedback
  Forward_Path : Subsystem  VariantControl=Forward
  Out1 : Outport  SampleTime=SampleTime

== system BMD_2_backup/FCS/Controller/roll_pitch_controller/PID Controller/Anti-windup ==
  preSat : Inport  SampleTime=SampleTime
  postSat : Inport  Port=2  SampleTime=SampleTime
  P : Inport  Port=3  SampleTime=SampleTime
  preInt : Inport  Port=4  SampleTime=SampleTime
  Upper Limit : Inport  Port=5  SampleTime=SampleTime
  Lower Limit : Inport  Port=6  SampleTime=SampleTime
  Back Calculation : Subsystem  VariantControl=BackCalculation
  Cont. Clamping Ideal : Subsystem  VariantControl=ContClampingIdeal
  Cont. Clamping Parallel : Subsystem  VariantControl=ContClampingParallel
  Disabled : Subsystem  VariantControl=Disabled
  Disc. Clamping Ideal : Subsystem  VariantControl=DiscClampingIdeal
  Disc. Clamping Parallel : Subsystem  VariantControl=DiscClampingParallel
  Passthrough : Subsystem  VariantControl=Passthrough
  Out1 : Outport  SampleTime=SampleTime

== system BMD_2_backup/FCS/Controller/roll_pitch_controller/PID Controller/D Gain ==
  err : Inport  SampleTime=SampleTime
  D Gain : Inport  Port=2  SampleTime=SampleTime
  Disabled : Subsystem  VariantControl=Disabled
  External Parameters : Subsystem  VariantControl=ExternalParameters
  Internal Parameters : Subsystem  VariantControl=InternalParameters
  Out1 : Outport  SampleTime=SampleTime

== system BMD_2_backup/FCS/Controller/roll_pitch_controller/PID Controller/External Derivative ==
  err : Inport  SampleTime=SampleTime
  ydot : Inport  Port=2  SampleTime=SampleTime
  Disabled : Subsystem  VariantControl=Disabled
  Error : Subsystem  VariantControl=ErrorSignal
  External Ydot : Subsystem  VariantControl=ExternalYdot
  Out1 : Outport  SampleTime=SampleTime

== system BMD_2_backup/FCS/Controller/roll_pitch_controller/PID Controller/Filter ==
  Reset : Inport  SampleTime=SampleTime
  U : Inport  Port=2  SampleTime=SampleTime
  N : Inport  Port=3  SampleTime=SampleTime
  D0in : Inport  Port=4  SampleTime=SampleTime
  Nout : Inport  Port=5  SampleTime=SampleTime
  Ts : Inport  Port=6  SampleTime=SampleTime
  Cont. Filter : Subsystem  VariantControl=ContFilter
  Cont. Filter Only : Subsystem  VariantControl=ContFilterOnly
  Differentiator : Subsystem  VariantControl=Differentiator
  Disabled : Subsystem  VariantControl=Disabled
  Disc. Backward Euler Filter : Subsystem  VariantControl=BackwardEulerFilter
  Disc. Backward Euler Filter Only : Subsystem  VariantControl=BackwardEulerFilterOnly
  Disc. Forward Euler Filter : Subsystem  VariantControl=ForwardEulerFilter
  Disc. Forward Euler Filter Only : Subsystem  VariantControl=ForwardEulerFilterOnly
  Disc. Trapezoidal Filter : Subsystem  VariantControl=TrapezoidalFilter
  Disc. Trapezoidal Filter Only : Subsystem  VariantControl=TrapezoidalFilterOnly
  Passthrough : Subsystem  VariantControl=Passthrough
  Y : Outport  SampleTime=SampleTime

== system BMD_2_backup/FCS/Controller/roll_pitch_controller/PID Controller/Filter ICs ==
  D0 : Inport  SampleTime=SampleTime
  Disabled : Subsystem  VariantControl=Disabled
  External IC : Subsystem  VariantControl=ExternalICs
  Internal IC - Differentiator : Subsystem  VariantControl=InternalICsDifferentiator
  Internal IC - Filter : Subsystem  VariantControl=InternalICsFilter
  Out1 : Outport  SampleTime=SampleTime

== system BMD_2_backup/FCS/Controller/roll_pitch_controller/PID Controller/I Gain ==
  err : Inport  SampleTime=SampleTime
  I Gain : Inport  Port=2  SampleTime=SampleTime
  Disabled : Subsystem  VariantControl=Disabled
  External Parameters : Subsystem  VariantControl=ExternalParameters
  Internal Parameters : Subsystem  VariantControl=InternalParameters
  Out1 : Outport  SampleTime=SampleTime

== system BMD_2_backup/FCS/Controller/roll_pitch_controller/PID Controller/Ideal P Gain ==
  In1 : Inport  SampleTime=SampleTime
  P Gain : Inport  Port=2  SampleTime=SampleTime
  External Parameters : Subsystem  VariantControl=ExternalParameters
  Internal Parameters : Subsystem  VariantControl=InternalParameters
  Passthrough : Subsystem  VariantControl=Disabled
  Out1 : Outport  SampleTime=SampleTime

== system BMD_2_backup/FCS/Controller/roll_pitch_controller/PID Controller/Ideal P Gain Fdbk ==
  In1 : Inport  SampleTime=SampleTime
  P Gain : Inport  Port=2  SampleTime=SampleTime
  Disabled : Subsystem  VariantControl=Disabled
  External Parameters : Subsystem  VariantControl=ExternalParameters
  Internal Parameters : Subsystem  VariantControl=InternalParameters
  Passthrough : Subsystem  VariantControl=Passthrough
  Out1 : Outport  SampleTime=SampleTime

== system BMD_2_backup/FCS/Controller/roll_pitch_controller/PID Controller/Integrator ==
  U : Inport  SampleTime=SampleTime
  I0in : Inport  Port=2  SampleTime=SampleTime
  Reset : Inport  Port=3  SampleTime=SampleTime
  Continuous : Subsystem  VariantControl=Continuous
  Disabled : Subsystem  VariantControl=Disabled
  Discrete : Subsystem  VariantControl=Discrete
  state : Outport  SampleTime=SampleTime
  out : Outport  Port=2  SampleTime=SampleTime

== system BMD_2_backup/FCS/Controller/roll_pitch_controller/PID Controller/Integrator ICs ==
  I0 : Inport  SampleTime=SampleTime
  Disabled : Subsystem  VariantControl=Disabled
  External IC : Subsystem  VariantControl=ExternalICs
  Internal IC : Subsystem  VariantControl=InternalICs
  Out1 : Outport  SampleTime=SampleTime

== system BMD_2_backup/FCS/Controller/roll_pitch_controller/PID Controller/N Copy ==
  N Gain : Inport  SampleTime=SampleTime
  Disabled : Subsystem  VariantControl=Disabled
  Disabled wSignal Specification : Subsystem  VariantControl=Disabled_SignalSpec
  External Parameters : Subsystem  VariantControl=ExternalParameters
  Internal Parameters : Subsystem  VariantControl=InternalParameters
  Out1 : Outport  SampleTime=SampleTime

== system BMD_2_backup/FCS/Controller/roll_pitch_controller/PID Controller/N Gain ==
  U : Inport  SampleTime=SampleTime
  N Gain : Inport  Port=2  SampleTime=SampleTime
  Disabled : Subsystem  VariantControl=Disabled
  External Parameters : Subsystem  VariantControl=ExternalParameters
  Internal Parameters : Subsystem  VariantControl=InternalParameters
  Passthrough : Subsystem  VariantControl=Passthrough
  Out1 : Outport  SampleTime=SampleTime

== system BMD_2_backup/FCS/Controller/roll_pitch_controller/PID Controller/P Copy ==
  P Gain : Inport  SampleTime=SampleTime
  Disabled : Subsystem  VariantControl=Disabled
  External Parameters Ideal : Subsystem  VariantControl=ExternalParamsIdeal
  Internal Parameters Ideal : Subsystem  VariantControl=InternalParamsIdeal
  Out1 : Outport  SampleTime=SampleTime

== system BMD_2_backup/FCS/Controller/roll_pitch_controller/PID Controller/PID Compensator Formula ==

== system BMD_2_backup/FCS/Controller/roll_pitch_controller/PID Controller/Parallel P Gain ==
  err : Inport  SampleTime=SampleTime
  P Gain : Inport  Port=2  SampleTime=SampleTime
  Disabled : Subsystem  VariantControl=Disabled
  External Parameters : Subsystem  VariantControl=ExternalParameters
  Internal Parameters : Subsystem  VariantControl=InternalParameters
  Passthrough : Subsystem  VariantControl=Passthrough
  Out1 : Outport  SampleTime=SampleTime

== system BMD_2_backup/FCS/Controller/roll_pitch_controller/PID Controller/Reset Signal ==
  Reset : Inport  SampleTime=SampleTime
  Disabled : Subsystem  VariantControl=Disabled
  External Reset : Subsystem  VariantControl=ExternalReset
  Out1 : Outport  SampleTime=SampleTime

== system BMD_2_backup/FCS/Controller/roll_pitch_controller/PID Controller/Saturation ==
  In1 : Inport  SampleTime=SampleTime
  Upper Limit : Inport  Port=2  SampleTime=SampleTime
  Lower Limit : Inport  Port=3  SampleTime=SampleTime
  Enabled : Subsystem  VariantControl=Enabled
  External : Subsystem  VariantControl=External
  Passthrough : Subsystem  VariantControl=Disabled
  Out1 : Outport  SampleTime=SampleTime

== system BMD_2_backup/FCS/Controller/roll_pitch_controller/PID Controller/Saturation Fdbk ==
  In1 : Inport  SampleTime=SampleTime
  Upper Limit : Inport  Port=2  SampleTime=SampleTime
  Lower Limit : Inport  Port=3  SampleTime=SampleTime
  Disabled : Subsystem  VariantControl=Disabled
  Enabled : Subsystem  VariantControl=Enabled
  External : Subsystem  VariantControl=External
  Passthrough : Subsystem  VariantControl=Passthrough
  Out1 : Outport  SampleTime=SampleTime

== system BMD_2_backup/FCS/Controller/roll_pitch_controller/PID Controller/Sum ==
  P : Inport  SampleTime=SampleTime
  I : Inport  Port=2  SampleTime=SampleTime
  D : Inport  Port=3  SampleTime=SampleTime
  Passthrough_I : Subsystem  VariantControl=Passthrough_I
  Passthrough_P : Subsystem  VariantControl=Passthrough_P
  Sum_PD : Subsystem  VariantControl=Sum_PD
  Sum_PI : Subsystem  VariantControl=Sum_PI
  Sum_PID : Subsystem  VariantControl=Sum_PID
  Out1 : Outport  SampleTime=SampleTime

== system BMD_2_backup/FCS/Controller/roll_pitch_controller/PID Controller/Sum Fdbk ==
  fromP : Inport  SampleTime=SampleTime
  fromState : Inport  Port=2  SampleTime=SampleTime
  fromD : Inport  Port=3  SampleTime=SampleTime
  Disabled : Subsystem  VariantControl=Disabled
  Enabled : Subsystem  VariantControl=Enabled
  Passthrough : Subsystem  VariantControl=Passthrough
  Out1 : Outport  SampleTime=SampleTime

== system BMD_2_backup/FCS/Controller/roll_pitch_controller/PID Controller/Tracking Mode ==
  uout : Inport  SampleTime=SampleTime
  TR : Inport  Port=2  SampleTime=SampleTime
  Disabled : Subsystem  VariantControl=Disabled
  Enabled : Subsystem  VariantControl=Enabled
  Out1 : Outport  SampleTime=SampleTime

== system BMD_2_backup/FCS/Controller/roll_pitch_controller/PID Controller/Tracking Mode Sum ==
  fromIgain : Inport  SampleTime=SampleTime
  fromTR : Inport  Port=2  SampleTime=SampleTime
  Passthrough : Subsystem  VariantControl=Passthrough
  Tracking Mode : Subsystem  VariantControl=TrackingMode
  preInt : Outport

== system BMD_2_backup/FCS/Controller/roll_pitch_controller/PID Controller/Tsamp - Integral ==
  U : Inport  SampleTime=SampleTime
  Ts : Inport  Port=2  SampleTime=SampleTime
  Disabled : Subsystem  VariantControl=Disabled
  External Ts : Subsystem  VariantControl=ExternalTs
  Passthrough : Subsystem  VariantControl=Passthrough
  TsSignalSpecification : Subsystem  VariantControl=Disabled_SignalSpec
  Out1 : Outport  SampleTime=SampleTime

== system BMD_2_backup/FCS/Controller/roll_pitch_controller/PID Controller/Tsamp - Ngain ==
  U : Inport  SampleTime=SampleTime
  Ts : Inport  Port=2  SampleTime=SampleTime
  External Ts : Subsystem  VariantControl=ExternalTs
  Passthrough : Subsystem  VariantControl=Passthrough
  Out1 : Outport  SampleTime=SampleTime

== system BMD_2_backup/FCS/Controller/roll_pitch_controller/PID Controller/postSat Signal ==
  feedback : Inport  SampleTime=SampleTime
  forward : Inport  Port=2  SampleTime=SampleTime
  Feedback_Path : Subsystem  VariantControl=Feedback
  Forward_Path : Subsystem  VariantControl=Forward
  Out1 : Outport  SampleTime=SampleTime

== system BMD_2_backup/FCS/Controller/roll_pitch_controller/PID Controller/preInt Signal ==
  preInt : Inport  SampleTime=SampleTime
  extAW : Inport  Port=2  SampleTime=SampleTime
  External PreInt : Subsystem  VariantControl=ExternalPreInt
  Internal PreInt : Subsystem  VariantControl=InternalPreInt
  Out1 : Outport  SampleTime=SampleTime

== system BMD_2_backup/FCS/Controller/roll_pitch_controller/PID Controller/preSat Signal ==
  feedback : Inport  SampleTime=SampleTime
  forward : Inport  Port=2  SampleTime=SampleTime
  Feedback_Path : Subsystem  VariantControl=Feedback
  Forward_Path : Subsystem  VariantControl=Forward
  Out1 : Outport  SampleTime=SampleTime
